simulink model "sfbp"  (Simulink 5.0)
settings: Solver=ode45  StartTime=0.0  StopTime=10000  RelTol=1e-3
settings Model: LastModifiedBy=Admin  RTWOptions="-aEnforceIntegerDowncast=1 -aExtMode=0 -aExtModeTesting=0 -aFoldNonRolledExpr=1 -aForceParamTrailComments=0 -aGenerateComments=1 -aGenerateReport=0 -aIgnoreCustomStorageClasses=1 -aIncDataTypeInIds=0 -aIncHierarchyInIds=0 -aInlineInvariantSignals=0 -aInlinedPrmAccess=\"Literals\" -aLocalBlockOutputs=1 -aLogVarNameModifier=\"rt_\" -aMaxRTWIdLen=31 -aPrefixModelToSubsysFcnNames=1 -aRTWVerbose=1 -aRollThreshold=5 -aShowEliminatedStatements=0"

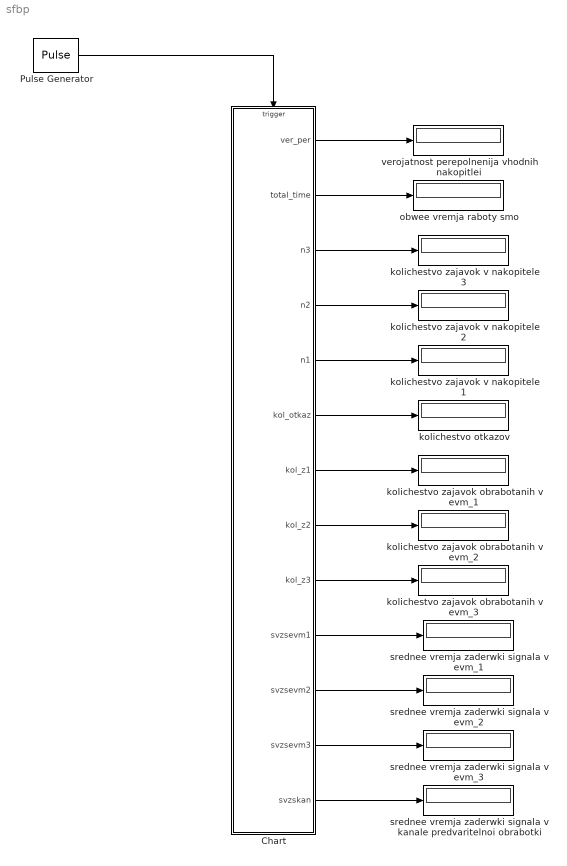
== system sfbp ==
  Chart : Stateflow chart
  Pulse Generator : DiscretePulseGenerator  PulseType=Time based  Period=1  PulseWidth=50
  kolichestvo otkazov : Display
  kolichestvo zajavok obrabotanih v evm_1 : Display
  kolichestvo zajavok obrabotanih v evm_2 : Display
  kolichestvo zajavok obrabotanih v evm_3 : Display
  kolichestvo zajavok v nakopitele 1 : Display
  kolichestvo zajavok v nakopitele 2 : Display
  kolichestvo zajavok v nakopitele 3 : Display
  obwee vremja raboty smo : Display
  srednee vremja zaderwki signala v evm_1 : Display
  srednee vremja zaderwki signala v evm_2 : Display
  srednee vremja zaderwki signala v evm_3 : Display
  srednee vremja zaderwki signala v kanale predvaritelnoi obrabotki : Display
  verojatnost perepolnenija vhodnih nakopitlei : Display
  wires:
  Pulse Generator/1 -> Chart/Trigger
  Chart/1(ver_per) -> verojatnost perepolnenija vhodnih nakopitlei/1
  Chart/2(total_time) -> obwee vremja raboty smo/1
  Chart/3(n3) -> kolichestvo zajavok v nakopitele 3/1
  Chart/4(n2) -> kolichestvo zajavok v nakopitele 2/1
  Chart/5(n1) -> kolichestvo zajavok v nakopitele 1/1
  Chart/6(kol_otkaz) -> kolichestvo otkazov/1
  Chart/7(kol_z1) -> kolichestvo zajavok obrabotanih v evm_1/1
  Chart/8(kol_z2) -> kolichestvo zajavok obrabotanih v evm_2/1
  Chart/9(kol_z3) -> kolichestvo zajavok obrabotanih v evm_3/1
  Chart/10(svzsevm1) -> srednee vremja zaderwki signala v evm_1/1
  Chart/11(svzsevm2) -> srednee vremja zaderwki signala v evm_2/1
  Chart/12(svzsevm3) -> srednee vremja zaderwki signala v evm_3/1
  Chart/13(svzskan) -> srednee vremja zaderwki signala v kanale predvaritelnoi obrabotki/1

== stateflow chart Chart ==
  state SMO/
    state Istochnik/ [parallel]
      state zaderwka/
      state vihod/
        entry:prihod=1;
        kolzajv++;
      state stopinng/
      vihod -> (junction 28) : /{Tmew=ml('round(unifrnd(5,15))');prihod=0;}
      zaderwka -> vihod
      (default) -> zaderwka : /kolzajv=0;
          | Tmew=0;
          | prihod=0;
      zaderwka -> zaderwka : [Tmew>0]/{Tmew--}
      (junction 28) -> zaderwka
      (junction 28) -> stopinng : [kolzajv==500]/
    state besknakop/ [parallel]
      state beskonechnakopitel/
      (default) -> beskonechnakopitel : /bocher=0;
      beskonechnakopitel -> beskonechnakopitel : [prihod==1]/{bocher++}
    state predvaritobrabotka/ [parallel]
      state vhod/
      state obrabotka/
      vhod -> (junction 42) : [bocher>0]/{Tobs=ml('round(unifrnd(7,13))')}
      obrabotka -> vhod : /{osv_kan0=1;}
      (default) -> vhod : /Tobs=0;
          | Tobssum=0;
      obrabotka -> obrabotka : [Tobs>0]/{Tobs--}
      (junction 48) -> obrabotka : /{bocher--;}
      (junction 42) -> (junction 48) : /{Tobssum+=Tobs}
    state vetvlenie/ [parallel]
      state raspredelenie/
      (junction 34) -> (junction 38) : /{n3++}
      (junction 35) -> (junction 29) : /{n2++}
      (junction 32) -> (junction 35) : [(raspr>2/3)&&(raspr<=1)]/
      raspredelenie -> (junction 37) : [osv_kan0==1]/
      (junction 30) -> (junction 35) : [(n2<n1)&&(n2<=n3)]/
      (junction 30) -> (junction 33) : [(n1<n3)&&(n1<=n2)]/
      (junction 30) -> (junction 34) : [(n3<=n1)&&(n3<n2)]/
      (junction 32) -> (junction 34) : [(raspr>1/3)&&(raspr<=2/3)]/
      (junction 51) -> (junction 32) : [(n2==n3)&&(n1==n2)]/{raspr=ml('unifrnd(0,1)')}
      (junction 33) -> (junction 36) : /{n1++}
      (junction 47) -> raspredelenie : [(n1==10)&&(n2==10)&&(n3==10)]/{kol_otkaz++}
      (default) -> raspredelenie : /kol_otkaz=0;
          | n1=0;n2=0;n3=0;
          | raspr=0;
      (junction 37) -> (junction 47) : /{osv_kan0=0;}
      (junction 38) -> (junction 39)
      (junction 36) -> (junction 39)
      (junction 29) -> (junction 39)
      (junction 39) -> raspredelenie
      (junction 51) -> (junction 30)
      (junction 32) -> (junction 33) : [(raspr>=0)&&(raspr<=1/3)]/
      (junction 47) -> (junction 51)
    state evm_1/ [parallel]
      state vhod1/
      state obsluwivanie1/
      vhod1 -> (junction 41) : [n1>0]/
      (junction 40) -> (junction 31) : [n1+n2+n3<25]/{Tobs1=33}
      (default) -> vhod1 : /Tobs1=0;
          | kol_z1=0;
          | Tobs1sum=0;
      obsluwivanie1 -> obsluwivanie1 : [Tobs1>0]/{Tobs1--}
      (junction 40) -> (junction 31) : [n1+n2+n3>=25]/{Tobs1=25}
      obsluwivanie1 -> vhod1 : /{kol_z1++}
      (junction 41) -> (junction 40) : /{n1--}
      (junction 31) -> obsluwivanie1 : /{Tobs1sum+=Tobs1}
    state evm_2/ [parallel]
      state vhod2/
      state obsluwivanie2/
      (default) -> vhod2 : /Tobs2=0;
          | kol_z2=0;
          | Tobs2sum=0;
      vhod2 -> (junction 43) : [n2>0]/
      (junction 43) -> (junction 44) : /{n2--}
      (junction 44) -> (junction 50) : [n1+n2+n3<25]/{Tobs2=33}
      (junction 44) -> (junction 50) : [n1+n2+n3>=25]/{Tobs2=25}
      obsluwivanie2 -> obsluwivanie2 : [Tobs2>0]/{Tobs2--}
      obsluwivanie2 -> vhod2 : /{kol_z2++}
      (junction 50) -> obsluwivanie2 : /{Tobs2sum+=Tobs2}
    state evm_3/ [parallel]
      state vhod3/
      state obsluwivanie3/
      vhod3 -> (junction 45) : [n3>0]/
      (junction 45) -> (junction 46) : /{n3--}
      (junction 46) -> (junction 49) : [n1+n2+n3<25]/{Tobs3=33}
      (junction 46) -> (junction 49) : [n1+n2+n3>=25]/{Tobs3=25}
      obsluwivanie3 -> obsluwivanie3 : [Tobs3>0]/{Tobs3--}
      obsluwivanie3 -> vhod3 : /{kol_z3++}
      (default) -> vhod3 : /kol_z3=0;
          | Tobs3=0;
          | Tobs3sum=0;
      (junction 49) -> obsluwivanie3 : /{Tobs3sum+=Tobs3}
    state statistica2/ [parallel]
      state stat2/
        exit:ver_per=kol_otkaz/kolzajv;
        exit:svzskan=Tobssum/kolzajv;
        exit:svzsevm1=Tobs1sum/kol_z1;
        exit:svzsevm2=Tobs2sum/kol_z2;
        exit:svzsevm3=Tobs3sum/kol_z3;
      (default) -> stat2 : /ver_per=0;
      stat2 -> stat2 : [kol_z1+kol_z2+kol_z3+kol_otkaz==500]/
    state statistica1/ [parallel]
      state stat1/
        entry:total_time++;
      (default) -> stat1 : /total_time=0;
      stat1 -> stat1 : [kol_z1+kol_z2+kol_z3+kol_otkaz<500]/
  data: Tmew local; bocher local; kolzajv local; prihod local; Tobs local; Tobs1 local; Tobs2 local; Tobs3 local; osv_kan0 local; ver_per output; total_time output; n3 output; n2 output; n1 output; kol_otkaz output; kol_z1 output; kol_z2 output; kol_z3 output; raspr local; Tobs1sum local; Tobs2sum local; Tobs3sum local; Tobssum local; svzsevm1 output; svzsevm2 output; svzsevm3 output; svzskan output
  events: event input RISING_EDGE_EVENT
